simulink model "nominal_control"  (R2024b)
settings: Solver=FixedStepAuto  StartTime=0.0  StopTime=10.0  FixedStep=T  RelTol=1e-3
settings Model: DataDictionary=wrapper2.sldd  Creator=maciej  LastModifiedBy=maciej

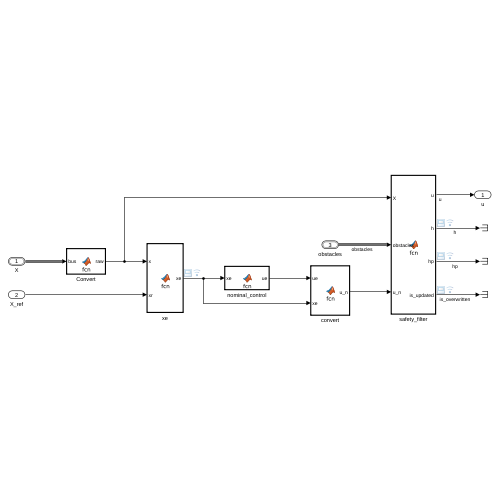
[thumbnail: Simulink's stored preview of the top-level diagram]
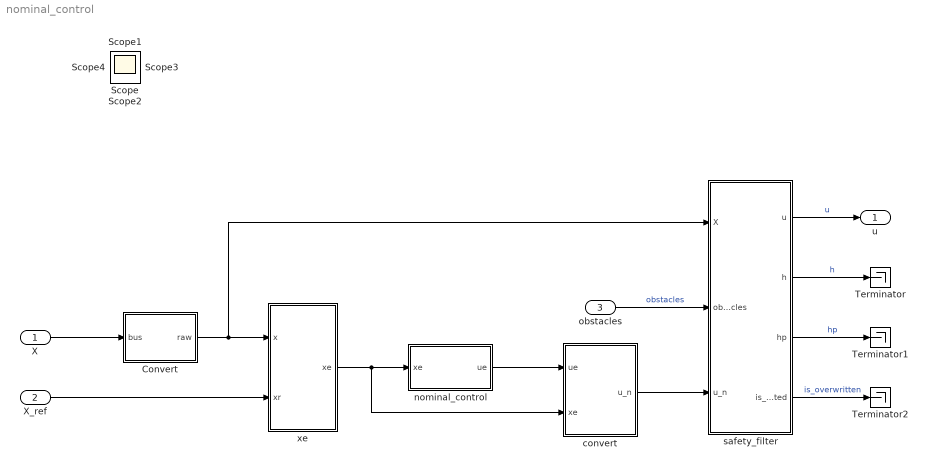
== system nominal_control ==
  X : Inport  OutDataTypeStr=Bus: EgoVehicle
  X_ref : Inport  Port=2  OutDataTypeStr=double  PortDimensions=[1, 6]
  obstacles : Inport  Port=3  OutDataTypeStr=Bus: Actors
  Convert : MATLAB Function  TreatAsAtomicUnit=on
  Terminator : Terminator
  Terminator1 : Terminator
  Terminator2 : Terminator
  convert : MATLAB Function  TreatAsAtomicUnit=on
  nominal_control : MATLAB Function  TreatAsAtomicUnit=on
  safety_filter : MATLAB Function  TreatAsAtomicUnit=on
  xe : MATLAB Function  TreatAsAtomicUnit=on
  u : Outport
  Scope{,1..4} (5 alike) : Scope
  wires:
  X/1 -> Convert/1(bus)
  Convert/1(raw) -> safety_filter/1(X), xe/1(x)
  xe/1(xe) -> convert/2(xe), nominal_control/1(xe)
  obstacles/1 -> safety_filter/2(obstacles)  "obstacles"
  nominal_control/1(ue) -> convert/1(ue)
  safety_filter/2(h) -> Terminator/1  "h"
  safety_filter/3(hp) -> Terminator1/1  "hp"
  convert/1(u_n) -> safety_filter/3(u_n)
  safety_filter/4(is_updated) -> Terminator2/1  "is_overwritten"
  safety_filter/1(u) -> u/1  "u"
  X_ref/1 -> xe/2(xr)

== matlab function nominal_control/nominal_control ==
  data: xe input; ue output
function ue = fcn(xe)
    K = ...
    [ ...
        0.1    0.0000    0.0000; ...
        0.0000   0.1     10.0995 ...
    ];

    ue = -K*xe;
end

== matlab function nominal_control/Convert ==
  data: bus input; raw output
function raw = fcn(bus)
    raw = [ ...
        bus.Position(1), ...
        bus.Position(2), ...
        deg2rad(bus.Yaw) ...
    ];
end

== matlab function nominal_control/safety_filter ==
  data: X input; u output; h output; obstacles input Bus: Actors; u_n input; hp output; is_updated output
function [u, h, hp, is_updated] = fcn(X, obstacles, u_n)
    x = X(1);
    y = X(2);
    theta = X(3);

    xo = 5;%obstacles.Actors(1).Position(1);
    yo = 0;%obstacles.Actors(1).Position(2);
    
    h = ((x - xo)^2 +(y - yo)^2 +  theta^2) - 1.5;
    dh = [2*x - 2*xo, 2*y - 2*yo, 2* theta];
    
    f = [0;0;0];
    g = [cos(theta) 0; sin(theta) 0; 0 1];
    
    q = @(ub)norm(ub-u_n)^2;
    x0 = u_n;
    A = -dh*g;
    b = dh*f + 1*h;
    options = optimoptions('fmincon', 'Algorithm', 'sqp', 'Display', 'off');
    u = fmincon(q, x0, A, b, [], [], [0.05 -1000], [], [], options);

    
    hp = dh*f + dh*g*u;

    is_updated = abs(norm(u_n) - norm(u)) > 0.01;
end

== matlab function nominal_control/xe ==
  data: x input; xe output; xr input
function xe = fcn(x, xr)
    c = cos(x(3));
    s = sin(x(3));
    dx = [xr(1) - x(1); xr(3) - x(2); xr(5) - x(3)];

    xe = [c s 0; -s c 0; 0 0 1] * dx;
end

== matlab function nominal_control/convert ==
  data: ue input; u_n output; xe input
function u_n = fcn(ue, xe)
    v  = cos(xe(3)) - ue(1);
    w = 0 - ue(2);

    u_n = [v, w]';
end
